simulink model "estimation"  (R2014b)
settings: Solver=ode1  StartTime=0.0  StopTime=20  FixedStep=Ts  RelTol=1e-3
InitFcn:
  | estimation_initfcn
libraries: aerolibutil x9
settings Model: Creator=wirnshofer  LastModifiedBy=benediktibk

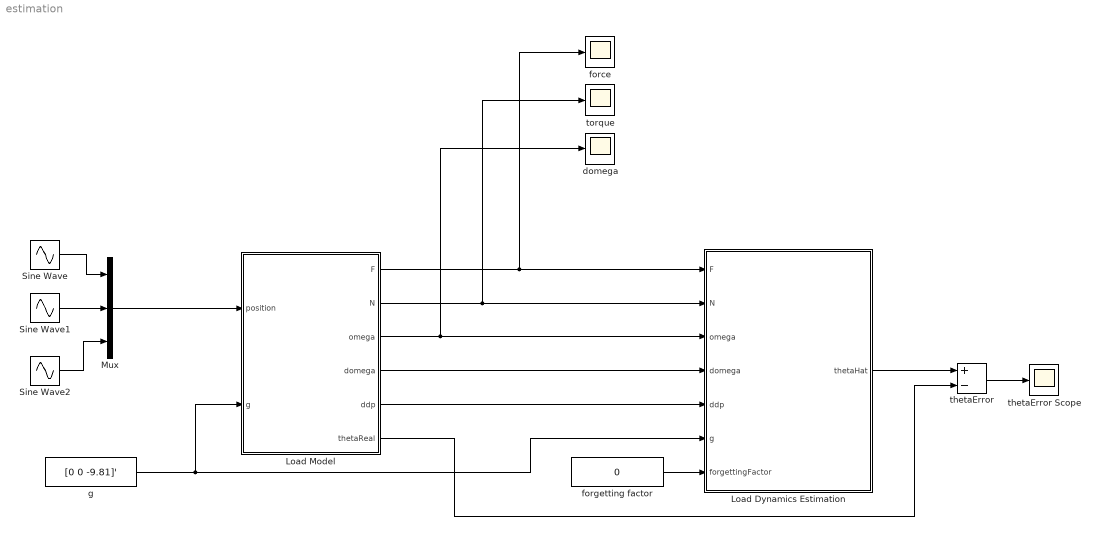
== system estimation ==
  Load Dynamics Estimation : MATLAB Function  TreatAsAtomicUnit=on
  Load Model : Subsystem  mask{mass=1, offsetGrasp=[2 1 4], Inertia=[1 0 0.5;0 3 0;0.5 0 4]}
      mask prompts: offsetGrasp "Grasping Offset"; Inertia "Inertia Matrix"
      mask DialogControl DescTextVar Prompt: Model
  Mux : Mux  Inputs=3
  Sine Wave : Sin  Frequency=0.5  SampleTime=0
  Sine Wave1 : Sin  Frequency=1.4  SampleTime=0
  Sine Wave2 : Sin  Frequency=0.7  SampleTime=0
  domega : Scope
      settings: YMin=0  YMax=0.8  SaveName=ScopeData3
  force : Scope
  forgetting factor : Constant  Value=0
  g : Constant  Value=[0 0 -9.81]'
  thetaError : Sum  Inputs=+-
  thetaError Scope : Scope
      settings: ShowLegends=on  YMin=1.25425  YMax=1.2595  SaveName=thetaError
  torque : Scope
  wires:
  Load Model/1(F) -> force/1, Load Dynamics Estimation/1(F)
  Load Model/2(N) -> torque/1, Load Dynamics Estimation/2(N)
  Sine Wave/1 -> Mux/1
  Sine Wave1/1 -> Mux/2
  Sine Wave2/1 -> Mux/3
  Mux/1 -> Load Model/1(position)
  Load Model/3(omega) -> domega/1, Load Dynamics Estimation/3(omega)
  Load Model/4(domega) -> Load Dynamics Estimation/4(domega)
  Load Model/5(ddp) -> Load Dynamics Estimation/5(ddp)
  g/1 -> Load Model/2(g), Load Dynamics Estimation/6(g)
  forgetting factor/1 -> Load Dynamics Estimation/7(forgettingFactor)
  Load Dynamics Estimation/1(thetaHat) -> thetaError/1
  Load Model/6(thetaReal) -> thetaError/2
  thetaError/1 -> thetaError Scope/1

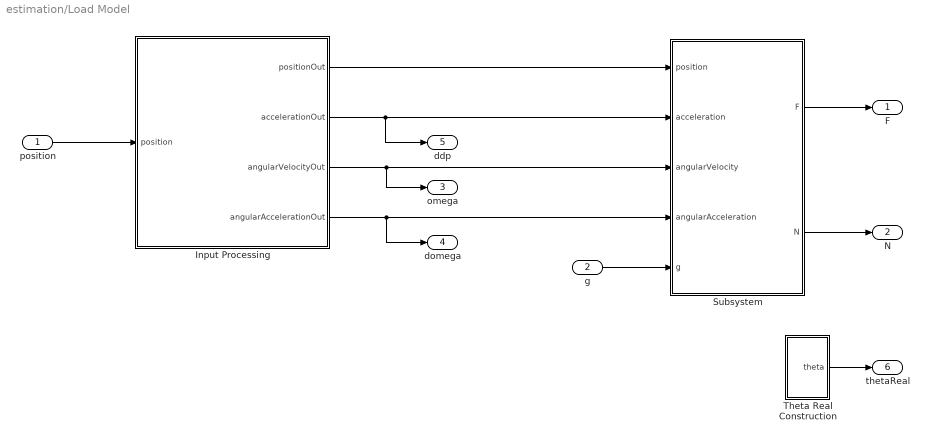
== system estimation/Load Model ==
  position : Inport
  g : Inport  Port=2
  Input Processing : Subsystem
  Subsystem : Subsystem
  Theta Real Construction : Subsystem
  F : Outport
  N : Outport  Port=2
  omega : Outport  Port=3
  domega : Outport  Port=4
  ddp : Outport  Port=5
  thetaReal : Outport  Port=6
  wires:
  position/1 -> Input Processing/1("position ")
  Input Processing/3(angularVelocityOut) -> omega/1, Subsystem/3(angularVelocity)
  Input Processing/4(angularAccelerationOut) -> domega/1, Subsystem/4(angularAcceleration)
  Input Processing/2(accelerationOut) -> ddp/1, Subsystem/2(acceleration)
  Theta Real Construction/1(theta) -> thetaReal/1
  Input Processing/1(positionOut) -> Subsystem/1(position)
  g/1 -> Subsystem/5(g)
  Subsystem/1(F) -> F/1
  Subsystem/2(N) -> N/1

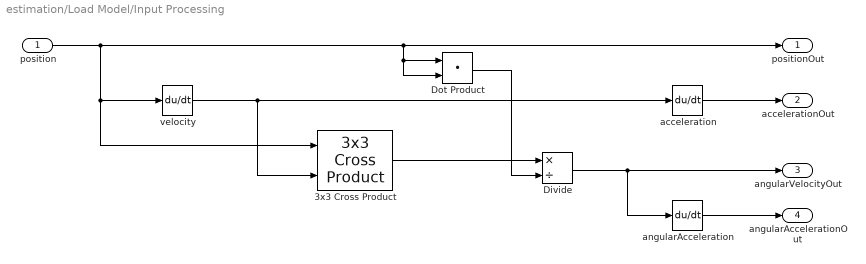
== system estimation/Load Model/Input Processing ==
  "position " : Inport
  3x3 Cross Product : aerolibutil/3x3 Cross Product
  Divide : Product  Inputs=*/
  Dot Product : DotProduct  InputSameDT=on  OutDataTypeStr=Inherit: Inherit via internal rule
  acceleration : Derivative
  angularAcceleration : Derivative
  velocity : Derivative
  positionOut : Outport
  accelerationOut : Outport  Port=2
  angularVelocityOut : Outport  Port=3
  angularAccelerationOut : Outport  Port=4
  wires:
  "position "/1 -> 3x3 Cross Product/1, velocity/1, positionOut/1, Dot Product/1, Dot Product/2
  angularAcceleration/1 -> angularAccelerationOut/1
  acceleration/1 -> accelerationOut/1
  velocity/1 -> 3x3 Cross Product/2, acceleration/1
  3x3 Cross Product/1 -> Divide/1
  Dot Product/1 -> Divide/2
  Divide/1 -> angularAcceleration/1, angularVelocityOut/1

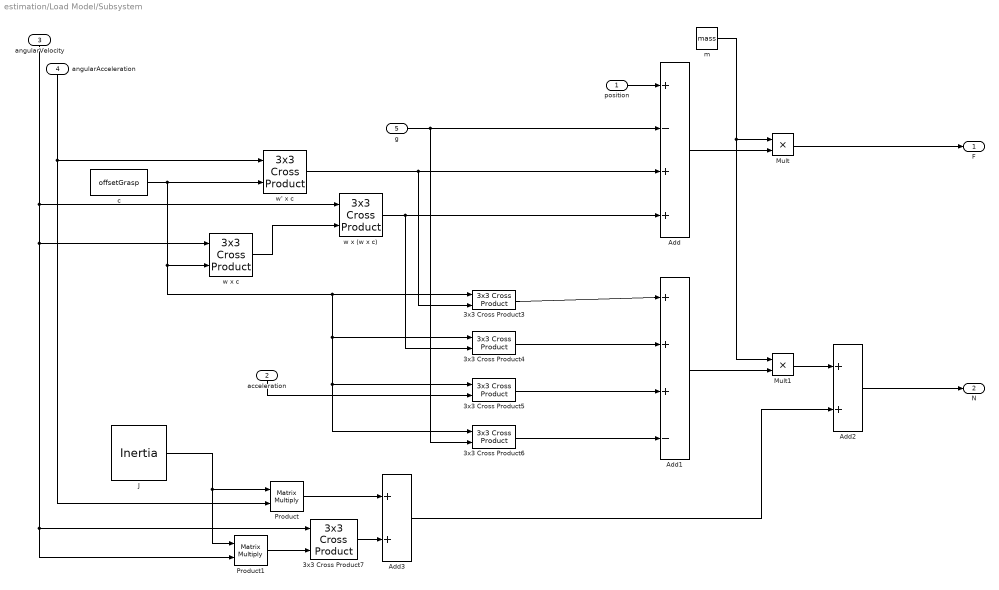
== system estimation/Load Model/Subsystem ==
  position : Inport
  acceleration : Inport  Port=2
  angularVelocity : Inport  Port=3
  angularAcceleration : Inport  Port=4
  g : Inport  Port=5
  3x3 Cross Product{3..7} (5 alike) : aerolibutil/3x3 Cross Product
  Add : Sum  Inputs=+-++
  Add1 : Sum  Inputs=+++-
  Add2 : Sum
  Add3 : Sum
  J : Constant  Value=Inertia  VectorParams1D=off
  Mult : Product  Inputs=**
  Mult1 : Product  Inputs=**
  Product : Product  Multiplication=Matrix(*)
  Product1 : Product  Multiplication=Matrix(*)
  c : Constant  Value=offsetGrasp
  m : Constant  Value=mass
  w x (w x c) : aerolibutil/3x3 Cross Product
  w x c : aerolibutil/3x3 Cross Product
  w' x c : aerolibutil/3x3 Cross Product
  F : Outport
  N : Outport  Port=2
  wires:
  acceleration/1 -> 3x3 Cross Product5/2
  angularVelocity/1 -> Product1/2, 3x3 Cross Product7/1, w x c/1, w x (w x c)/1
  angularAcceleration/1 -> Product/2, w' x c/1
  Product1/1 -> 3x3 Cross Product7/2
  Mult/1 -> F/1
  m/1 -> Mult1/1, Mult/1
  w' x c/1 -> Add/3, 3x3 Cross Product3/2
  Add2/1 -> N/1
  3x3 Cross Product3/1 -> Add1/1
  Add3/1 -> Add2/2
  w x c/1 -> w x (w x c)/2
  3x3 Cross Product5/1 -> Add1/3
  w x (w x c)/1 -> 3x3 Cross Product4/2, Add/4
  3x3 Cross Product6/1 -> Add1/4
  Product/1 -> Add3/1
  J/1 -> Product1/1, Product/1
  3x3 Cross Product7/1 -> Add3/2
  3x3 Cross Product4/1 -> Add1/2
  Add1/1 -> Mult1/2
  Add/1 -> Mult/2
  g/1 -> 3x3 Cross Product6/2, Add/2
  Mult1/1 -> Add2/1
  c/1 -> w x c/2, 3x3 Cross Product4/1, 3x3 Cross Product6/1, 3x3 Cross Product5/1, 3x3 Cross Product3/1, w' x c/2
  position/1 -> Add/1

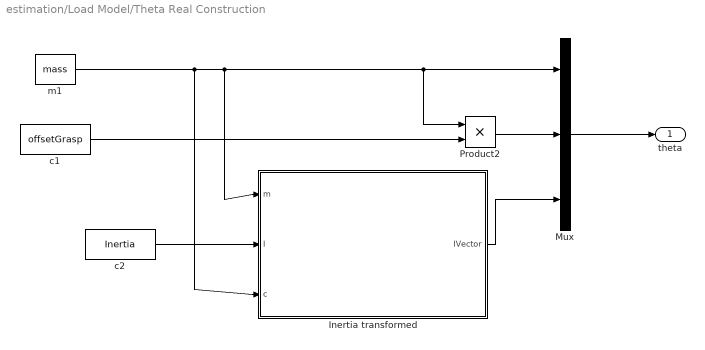
== system estimation/Load Model/Theta Real Construction ==
  Inertia transformed : MATLAB Function  TreatAsAtomicUnit=on
  Mux : Mux  Inputs=3
  Product2 : Product
  c1 : Constant  Value=offsetGrasp
  c2 : Constant  Value=Inertia
  m1 : Constant  Value=mass
  theta : Outport
  wires:
  m1/1 -> Inertia transformed/3(c), Inertia transformed/1(m), Product2/1, Mux/1
  c1/1 -> Product2/2
  Product2/1 -> Mux/2
  Mux/1 -> theta/1
  Inertia transformed/1(IVector) -> Mux/3
  c2/1 -> Inertia transformed/2(I)

== matlab function estimation/Load Dynamics Estimation ==
  data: F input; thetaHat output; N input; omega input; domega input; ddp input; g input; forgettingFactor input
function thetaHat = fcn(F,N,omega,domega,ddp,g,forgettingFactor)
persistent thetaHatPrevious PPrevious initializationNecessary;

if isempty(initializationNecessary)
    initializationNecessary = 1;
end

% calculate linear relation Phi between the estimates and the input
omegaCross = crossMatrix(omega);
domegaCross = crossMatrix(domega);
omegaDot = dotMatrix(omega);
domegaDot = dotMatrix(domega);
h = [F;N];
Phi = [ddp-g , domegaCross+omegaCross*omegaCross, zeros(3,6) ; zeros(3,1) , crossMatrix(g-ddp) , domegaDot+omegaCross*omegaDot];

% intialize persisent variables
if initializationNecessary == 1 || isempty(PPrevious)
    PPrevious = inv(Phi'*Phi);
    thetaHatPrevious = PPrevious*Phi'*h;
    thetaHat = thetaHatPrevious;
    initializationNecessary = 0;
    return;
end    

% check for invalid values in the current state
if any(any(isnan(PPrevious)))
    initializationNecessary = 1;
    thetaHat = thetaHatPrevious;
    return;  
end    

KInternal = eye(6)+Phi*PPrevious*Phi';
KInternalInv = inv(KInternal);

% check for invalid values in the current estimation step
if calculateConditionDistance(KInternal, KInternalInv) > 1e20
    initializationNecessary = 1;
    thetaHat = thetaHatPrevious;
    return;  
end

% calculate improved estimation
K = PPrevious*Phi'*KInternalInv;
PNew = (eye(10)-K*Phi)*PPrevious;
P = (1 - forgettingFactor)*PNew + forgettingFactor*PPrevious;
thetaHatNew = thetaHatPrevious+K*(h-Phi*thetaHatPrevious);
thetaHat = (1 - forgettingFactor)*thetaHatNew + forgettingFactor*thetaHatPrevious;
PPrevious = P;
thetaHatPrevious = thetaHat;

== matlab function estimation/Load Model/Theta Real Construction/Inertia transformed ==
  data: IVector output; m input; I input; c input
function IVector = transformInertia(m,I,c)

ITransformed = I + m*((c'*c)*eye(3) - (c*c'));
IVector = [ITransformed(1,1:3)';ITransformed(2,2:3)';ITransformed(3,3)];
